simulink model "Practica1"  (R2023a)
settings: Solver=VariableStepAuto  StartTime=0.0  StopTime=50  RelTol=1e-3
model workspace (MAT data in the model file):
  L1 = 0.3
  L2 = 0.25
  M1 = 0.2
  M2 = 0.1
  g = 9.81
settings Model: Creator=mluser

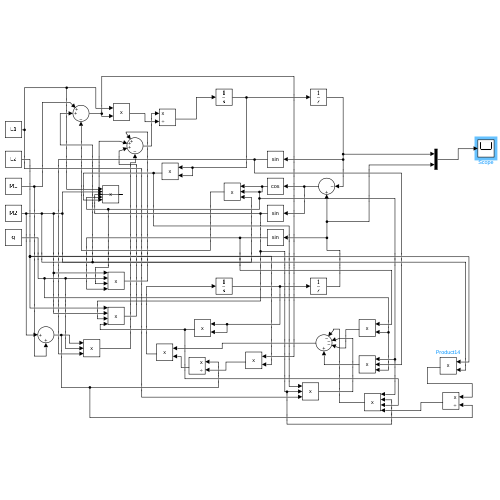
[thumbnail: Simulink's stored preview of the top-level diagram]
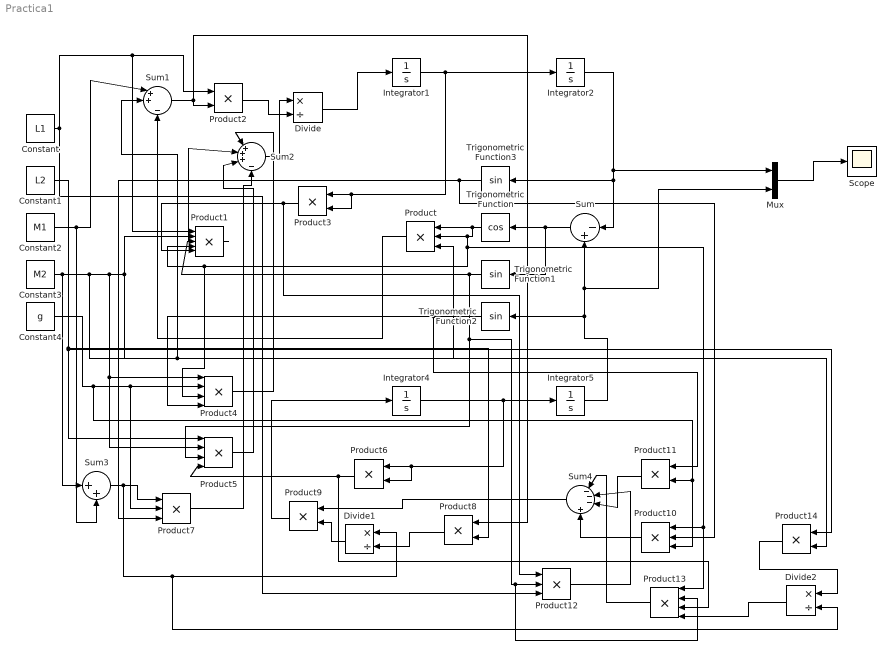
== system Practica1 ==
  Constant : Constant  Value=L1
  Constant1 : Constant  Value=L2
  Constant2 : Constant  Value=M1
  Constant3 : Constant  Value=M2
  Constant4 : Constant  Value=g
  Divide : Product  Inputs=*/
  Divide1 : Product  Inputs=*/
  Divide2 : Product  Inputs=*/
  Integrator1 : Integrator
  Integrator2 : Integrator
  Integrator4 : Integrator
  Integrator5 : Integrator  InitialCondition=35
  Mux : Mux  Inputs=2
  Product{,7,10,12} (4 alike) : Product  Inputs=3
  Product1 : Product  Inputs=5
  Product{2..3,6,8..9,11,14} (7 alike) : Product
  Product13 : Product  Inputs=4
  Product4 : Product  Inputs=4
  Product5 : Product  Inputs=4
  Scope : Scope
  Sum : Sum  Inputs=|-+
  Sum1 : Sum  Inputs=|++|-
  Sum2 : Sum  Inputs=|+++|-
  Sum3 : Sum  Inputs=|++
  Sum4 : Sum  Inputs=|---|+
  Trigonometric Function : Trigonometry  Operator=cos
  Trigonometric Function1 : Trigonometry
  Trigonometric Function2 : Trigonometry
  Trigonometric Function3 : Trigonometry
  wires:
  Trigonometric Function/1 -> Product13/1, Product10/1, Product4/3, Product1/4, Product/2, Product/1
  Sum/1 -> Trigonometric Function1/1, Trigonometric Function/1
  Constant3/1 -> Product14/2, Product5/2, Product4/1, Product1/2, Product/3, Sum1/2, Sum3/1
  Constant2/1 -> Sum1/1, Sum3/2
  Integrator1/1 -> Product3/2, Product3/1, Integrator2/1
  Integrator4/1 -> Product6/2, Product6/1, Integrator5/1
  Product/1 -> Sum1/3
  Sum1/1 -> Product2/2, Product8/1
  Constant/1 -> Product1/1, Product2/1, Product12/3
  Product2/1 -> Divide/2
  Trigonometric Function1/1 -> Product13/2, Product12/2, Product5/3, Product1/3
  Integrator5/1 -> Trigonometric Function2/1, Mux/2, Sum/2
  Integrator2/1 -> Trigonometric Function3/1, Sum/1, Mux/1
  Product3/1 -> Product12/1, Product1/5
  Constant4/1 -> Product11/2, Product10/3, Product7/2, Product4/2
  Divide/1 -> Integrator1/1
  Sum2/1 -> Divide/1
  Trigonometric Function2/1 -> Product11/1, Product4/4
  Product1/1 -> Sum2/2
  Product4/1 -> Sum2/1
  Constant1/1 -> Product14/1, Product5/1, Product8/2
  Product6/1 -> Product13/3, Product5/4
  Product5/1 -> Sum2/3
  Sum3/1 -> Divide2/2, Divide1/1, Product7/1
  Trigonometric Function3/1 -> Product10/2, Product7/3
  Product7/1 -> Sum2/4
  Product8/1 -> Divide1/2
  Divide1/1 -> Product9/2
  Product9/1 -> Integrator4/1
  Sum4/1 -> Product9/1
  Product10/1 -> Sum4/4
  Product11/1 -> Sum4/3
  Product12/1 -> Sum4/2
  Product13/1 -> Sum4/1
  Divide2/1 -> Product13/4
  Product14/1 -> Divide2/1
  Mux/1 -> Scope/1
